simulink model "sampleModel1978"  (R2023a)
settings: Solver=VariableStepAuto  StartTime=0.0  StopTime=10.0  RelTol=1e-3
libraries: hdlsllib x7, simulink x1
settings Model: Creator=user1  LastModifiedBy=user1

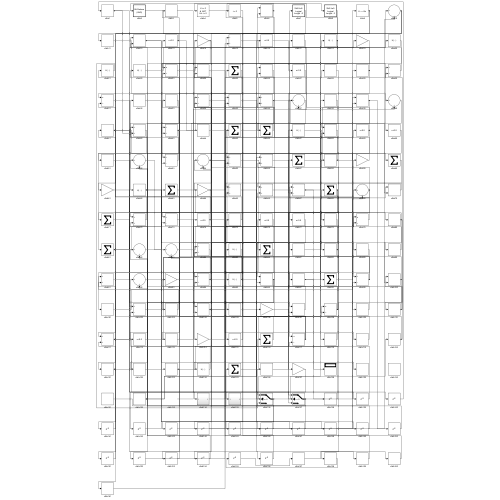
[thumbnail: Simulink's stored preview of the top-level diagram]
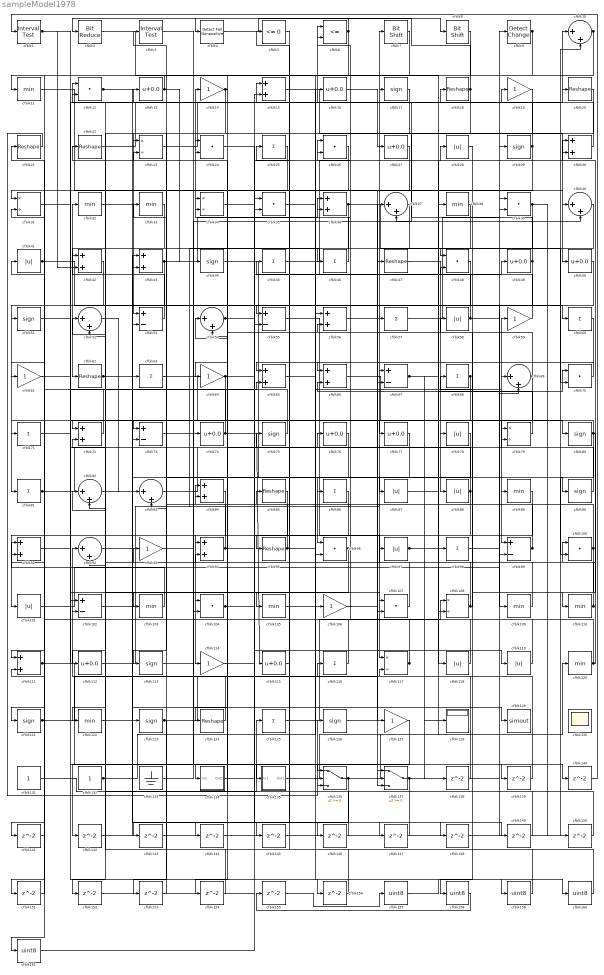
== system sampleModel1978 ==
  cfblk1 : hdlsllib/Logic and Bit Operations/Interval Test  IntervalClosedRight=on  uplimit=0.5  IntervalClosedLeft=on  lowlimit=-0.5  OutDataTypeStr=boolean
  cfblk{10,37,40,52,54,69,82..83,92} (9 alike) : Sum  Inputs=|++
  cfblk{12,24,26,35,39,48,70,96,100,104,107} (11 alike) : DotProduct  OutDataTypeStr=Inherit: Inherit via internal rule
  cfblk{28,41,58,78,87..88,97,101,118..119} (10 alike) : Abs  SaturateOnIntegerOverflow=off
  cfblk{53,55,67,73,99,102} (6 alike) : Sum  Inputs=+-
  cfblk{11,32..33,38,89,103,105,109..110,120,122} (11 alike) : MinMax
  cfblk{14,19,59,61,64,93,106,114,127} (9 alike) : Gain
  cfblk{23,31,34,79,108,117} (6 alike) : Product  Inputs=*/  RndMeth=Zero  SaturateOnIntegerOverflow=on
  cfblk{15,30,36,42..43,56,65..66,72,84,91,94,111} (13 alike) : Sum
  cfblk{13,16,27,49..50,74,76..77,112,115} (10 alike) : Bias  Bias=0.0  SaturateOnIntegerOverflow=off
  cfblk{17,29,44,51,75,80,90,113,121,123,126} (11 alike) : Signum
  cfblk{25,45..46,57,60,63,68,71,81,86,98,116,125} (13 alike) : Sum  Inputs=+
  cfblk{18,20..22,47,62,85,95,124} (9 alike) : Reshape
  cfblk128 : Display
  cfblk129 : ToWorkspace  VariableName=simout  SaveFormat=Timeseries  SampleTime=-1
  cfblk130 : Scope
      settings: Floating=on
  cfblk131 : Constant  SampleTime=-1
  cfblk132 : Constant  SampleTime=-1
  cfblk133 : Ground
  cfblk134 : Subsystem
      settings: LibrarySourceBlock=|
      | hdlsllib/Ports &
      | Subsystems/Subsystem
  cfblk135 : Subsystem
      settings: LibrarySourceBlock=|
      | hdlsllib/Ports &
      | Subsystems/Subsystem
  cfblk136 : Switch  SaturateOnIntegerOverflow=off  InputSameDT=off
  cfblk137 : Switch  SaturateOnIntegerOverflow=off  InputSameDT=off
  cfblk{138..156} (19 alike) : Delay  SampleTime=1
  cfblk{157..161} (5 alike) : DataTypeConversion  OutDataTypeStr=uint8  SaturateOnIntegerOverflow=off  RndMeth=Floor
  cfblk2 : hdlsllib/Logic and Bit Operations/Bit Reduce  mode=AND
  cfblk3 : hdlsllib/Logic and Bit Operations/Interval Test  IntervalClosedRight=on  uplimit=0.5  IntervalClosedLeft=on  lowlimit=-0.5  OutDataTypeStr=boolean
  cfblk4 : hdlsllib/Logic and Bit Operations/Detect Fall Nonpositive  vinit=0  OutDataTypeStr=boolean
  cfblk5 : hdlsllib/Logic and Bit Operations/Compare To Zero  relop=<=  OutDataTypeStr=boolean
  cfblk6 : RelationalOperator  Operator=<=  OutDataTypeStr=boolean  InputSameDT=off
  cfblk7 : hdlsllib/Logic and Bit Operations/Bit Shift  mode=Shift Left Logical  N=0
  cfblk8 : hdlsllib/Logic and Bit Operations/Bit Shift  mode=Shift Left Logical  N=0
  cfblk9 : simulink/Logic and Bit Operations/Detect Change  vinit=0  OutDataTypeStr=boolean
      settings: LibrarySourceBlock=|
      | hdlsllib/Logic and Bit
      | Operations/Detect
      | Change
  wires:
  cfblk108/1 -> cfblk7/1, cfblk58/1, cfblk82/2
  cfblk85/1 -> cfblk114/1
  cfblk46/1 -> cfblk14/1
  cfblk90/1 -> cfblk59/1
  cfblk40/1 -> cfblk92/1
  cfblk52/1 -> cfblk83/1
  cfblk44/1 -> cfblk96/1
  cfblk50/1 -> cfblk55/1
  cfblk42/1 -> cfblk81/1
  cfblk133/1 -> cfblk74/1
  cfblk125/1 -> cfblk108/1
  cfblk30/1 -> cfblk18/1
  cfblk112/1 -> cfblk26/1
  cfblk47/1 -> cfblk88/1
  cfblk117/1 -> cfblk21/1, cfblk12/2, cfblk85/1
  cfblk122/1 -> cfblk123/1
  cfblk79/1 -> cfblk17/1
  cfblk55/1 -> cfblk117/1
  cfblk131/1 -> cfblk125/1
  cfblk56/1 -> cfblk127/1
  cfblk39/1 -> cfblk62/1, cfblk150/1
  cfblk15/1 -> cfblk50/1
  cfblk43/1 -> cfblk51/1, cfblk36/1
  cfblk74/1 -> cfblk115/1, cfblk31/2
  cfblk16/1 -> cfblk27/1
  cfblk87/1 -> cfblk70/1
  cfblk113/1 -> cfblk76/1
  cfblk21/1 -> cfblk126/1
  cfblk33/1 -> cfblk72/1
  cfblk92/1 -> cfblk56/1
  cfblk102/1 -> cfblk67/1
  cfblk53/1 -> cfblk32/1
  cfblk5/1 -> cfblk95/1
  cfblk77/1 -> cfblk113/1
  cfblk19/1 -> cfblk53/1
  cfblk89/1 -> cfblk101/1
  cfblk126/1 -> cfblk47/1
  cfblk100/1 -> cfblk34/1, cfblk158/1
  cfblk94/1 -> cfblk33/1, cfblk137/2
  cfblk63/1 -> cfblk98/1
  cfblk111/1 -> cfblk134/1(In1), cfblk79/2
  cfblk26/1 -> cfblk61/1
  cfblk73/1 -> cfblk90/1
  cfblk48/1 -> cfblk92/2
  cfblk75/1 -> cfblk52/1
  cfblk88/1 -> cfblk97/1, cfblk34/2
  cfblk124/1 -> cfblk13/1
  cfblk58/1 -> cfblk60/1, cfblk36/2
  cfblk119/1 -> cfblk56/2
  cfblk13/1 -> cfblk11/1, cfblk44/1
  cfblk132/1 -> cfblk106/1, cfblk42/1, cfblk16/1
  cfblk62/1 -> cfblk148/1, cfblk149/1
  cfblk45/1 -> cfblk28/1
  cfblk18/1 -> cfblk2/1, cfblk37/2, cfblk122/1
  cfblk136/1 -> cfblk38/1, cfblk143/1
  cfblk37/1 -> cfblk46/1
  cfblk22/1 -> cfblk19/1
  cfblk7/1 -> cfblk105/1
  cfblk103/1 -> cfblk91/1
  cfblk70/1 -> cfblk65/1
  cfblk11/1 -> cfblk40/1
  cfblk14/1 -> cfblk73/1, cfblk54/2
  cfblk51/1 -> cfblk77/1
  cfblk71/1 -> cfblk135/1(In1)
  cfblk110/1 -> cfblk30/1, cfblk24/1
  cfblk114/1 -> cfblk26/2
  cfblk66/1 -> cfblk99/1
  cfblk6/1 -> cfblk4/1, cfblk136/2
  cfblk96/1 -> cfblk112/1, cfblk152/1
  cfblk121/1 -> cfblk116/1, cfblk151/1
  cfblk109/1 -> cfblk68/1
  cfblk9/1 -> cfblk31/1, cfblk161/1
  cfblk81/1 -> cfblk43/1, cfblk65/2
  cfblk135/1(Out1) -> cfblk120/1
  cfblk20/1 -> cfblk43/2
  cfblk17/1 -> cfblk23/1
  cfblk83/1 -> cfblk57/1
  cfblk99/1 -> cfblk84/1, cfblk24/2
  cfblk57/1 -> cfblk9/1
  cfblk49/1 -> cfblk94/1, cfblk12/1
  cfblk4/1 -> cfblk8/1
  cfblk91/1 -> cfblk15/1
  cfblk59/1 -> cfblk5/1
  cfblk23/1 -> cfblk10/1
  cfblk98/1 -> cfblk39/2
  cfblk107/1 -> cfblk6/1
  cfblk101/1 -> cfblk29/1
  cfblk41/1 -> cfblk109/1, cfblk156/1
  cfblk93/1 -> cfblk40/2
  cfblk78/1 -> cfblk104/1
  cfblk72/1 -> cfblk41/1
  cfblk120/1 -> cfblk75/1, cfblk100/1
  cfblk95/1 -> cfblk69/1, cfblk84/2
  cfblk54/1 -> cfblk89/1, cfblk96/2
  cfblk28/1 -> cfblk48/1
  cfblk115/1 -> cfblk45/1
  cfblk64/1 -> cfblk48/2, cfblk121/1
  cfblk69/1 -> cfblk22/1, cfblk66/2, cfblk137/3
  cfblk137/1 -> cfblk99/2, cfblk136/3
  cfblk106/1 -> cfblk137/1
  cfblk82/1 -> cfblk63/1
  cfblk38/1 -> cfblk53/2
  cfblk61/1 -> cfblk136/1
  cfblk67/1 -> cfblk49/1, cfblk128/1
  cfblk34/1 -> cfblk86/1
  cfblk25/1 -> cfblk103/1
  cfblk123/1 -> cfblk37/1, cfblk153/1
  cfblk27/1 -> cfblk67/2
  cfblk97/1 -> cfblk30/2, cfblk138/1
  cfblk134/1(Out1) -> cfblk79/1
  cfblk80/1 -> cfblk110/1, cfblk78/1, cfblk100/2
  cfblk12/1 -> cfblk129/1, cfblk80/1
  cfblk1/1 -> cfblk102/1, cfblk42/2
  cfblk31/1 -> cfblk107/1
  cfblk2/1 -> cfblk118/1
  cfblk32/1 -> cfblk87/1
  cfblk68/1 -> cfblk71/1, cfblk107/2
  cfblk8/1 -> cfblk111/1
  cfblk10/1 -> cfblk104/2, cfblk108/2, cfblk64/1
  cfblk24/1 -> cfblk119/1
  cfblk104/1 -> cfblk20/1, cfblk146/1
  cfblk116/1 -> cfblk93/1
  cfblk36/1 -> cfblk70/2, cfblk145/1
  cfblk29/1 -> cfblk6/2, cfblk124/1
  cfblk60/1 -> cfblk66/1
  cfblk118/1 -> cfblk3/1
  cfblk138/1 -> cfblk117/2
  cfblk3/1 -> cfblk139/1
  cfblk139/1 -> cfblk94/2
  cfblk65/1 -> cfblk140/1
  cfblk140/1 -> cfblk1/1
  cfblk84/1 -> cfblk141/1
  cfblk141/1 -> cfblk91/2
  cfblk127/1 -> cfblk142/1
  cfblk142/1 -> cfblk73/2
  cfblk143/1 -> cfblk69/2
  cfblk76/1 -> cfblk144/1
  cfblk144/1 -> cfblk15/2
  cfblk145/1 -> cfblk10/2
  cfblk146/1 -> cfblk52/2
  cfblk105/1 -> cfblk147/1
  cfblk147/1 -> cfblk54/1
  cfblk148/1 -> cfblk39/1
  cfblk149/1 -> cfblk82/1
  cfblk150/1 -> cfblk23/2
  cfblk151/1 -> cfblk111/2
  cfblk152/1 -> cfblk55/2
  cfblk153/1 -> cfblk83/2
  cfblk86/1 -> cfblk154/1
  cfblk154/1 -> cfblk72/2
  cfblk156/1 -> cfblk102/2
  cfblk155/1 -> cfblk157/1
  cfblk158/1 -> cfblk155/1
  cfblk35/1 -> cfblk159/1
  cfblk159/1 -> cfblk25/1
  cfblk157/1 -> cfblk160/1
  cfblk160/1 -> cfblk35/1
  cfblk161/1 -> cfblk35/2

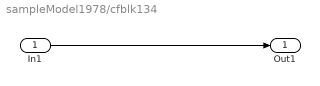
== system sampleModel1978/cfblk134 ==
  In1 : Inport
  Out1 : Outport
  wires:
  In1/1 -> Out1/1

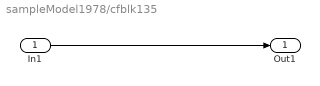
== system sampleModel1978/cfblk135 ==
  In1 : Inport
  Out1 : Outport
  wires:
  In1/1 -> Out1/1
